simulink model "quadrotor_model"  (R2021a)
settings: Solver=VariableStepAuto  StartTime=0.0  StopTime=20  RelTol=1e-1
values from neighbouring files (symbols this model uses):
  X = [X realx(index)]    [Plot_drone_3D.m]    (also in Plot_drone_3D_sub.m)
  Y = [Y realy(index)]    [Plot_drone_3D.m]    (also in Plot_drone_3D_sub.m)
  Z = [Z realz(index)]    [Plot_drone_3D.m]    (also in Plot_drone_3D_sub.m)
undefined symbols (not defined in the file or in its folder): Discrete, Time
libraries: sm_lib x6, vrlib x2, sharedtransform x2, aerolibutil x2, nesl_utility x1, dspmtrx3 x1, ctrlSharedLib x1
settings Model: EnablePacing=on  PacingRate=10  Creator=amejiyopakapak  LastModifiedBy=user

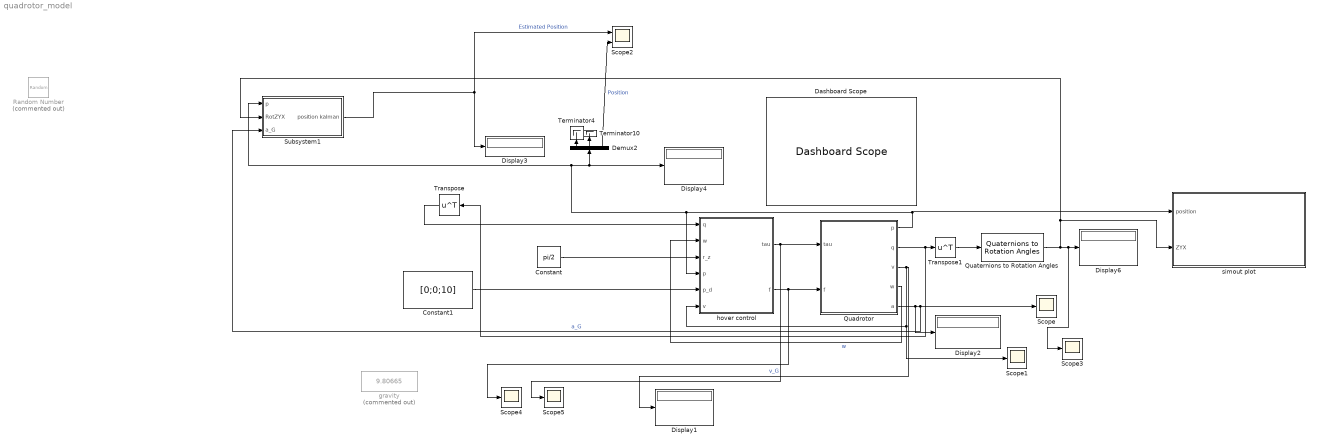
== system quadrotor_model ==
  Constant : Constant  Value=pi/2
  Constant1 : Constant  Value=[0;0;10]
  Dashboard Scope : DashboardScope
  Demux2 : Demux  Outputs=3
  Display{1..4,6} (5 alike) : Display
  Quadrotor : Subsystem
  Quaternions to Rotation Angles : sharedtransform/Quaternions to Rotation Angles  rotationOrder=ZYX  aMode=aMode
      settings: SourceProductBaseCode=AE,PW,DR,MT,UV,VE
  Random Number : RandomNumber  Commented=on  SampleTime=0.1
  Scope{,1,3..5} (5 alike) : Scope
  Scope2 : Scope  NumInputPorts=2
  Subsystem1 : Subsystem
  Terminator10 : Terminator
  Terminator4 : Terminator
  Transpose : Math  Operator=transpose  SaturateOnIntegerOverflow=on
  Transpose1 : Math  Operator=transpose  SaturateOnIntegerOverflow=on
  gravity : Constant  Commented=on  Value=9.80665
  hover control : Subsystem  mask{mass=1}
  simout plot : Subsystem
  wires:
  Quadrotor/5(a) -> Subsystem1/3(a_G), Scope/1, Display2/1  "a_G"
  Constant/1 -> hover control/3(r_z)
  Quadrotor/3(v) -> hover control/6(v), Scope1/1, Display1/1  "v_G"
  Quadrotor/2(q) -> Transpose/1, Transpose1/1
  hover control/1(tau) -> Quadrotor/1(tau), Scope5/1
  Quadrotor/4(w) -> hover control/2(w)  "w"
  Transpose/1 -> hover control/1(q)
  Quaternions to Rotation Angles/1 -> simout plot/2(ZYX), Subsystem1/2(RotZYX), Display6/1, Scope3/1
  Transpose1/1 -> Quaternions to Rotation Angles/1
  Constant1/1 -> hover control/5(p_d)
  hover control/2(f) -> Scope4/1, Quadrotor/2(f)
  Quadrotor/1(p) -> simout plot/1(position), Subsystem1/1(p), Demux2/1, Display4/1, hover control/4(p)
  Demux2/3 -> Scope2/2  "Position"
  Demux2/1 -> Terminator4/1
  Demux2/2 -> Terminator10/1
  Subsystem1/1(position kalman) -> Scope2/1, Display3/1  "Estimated Position"

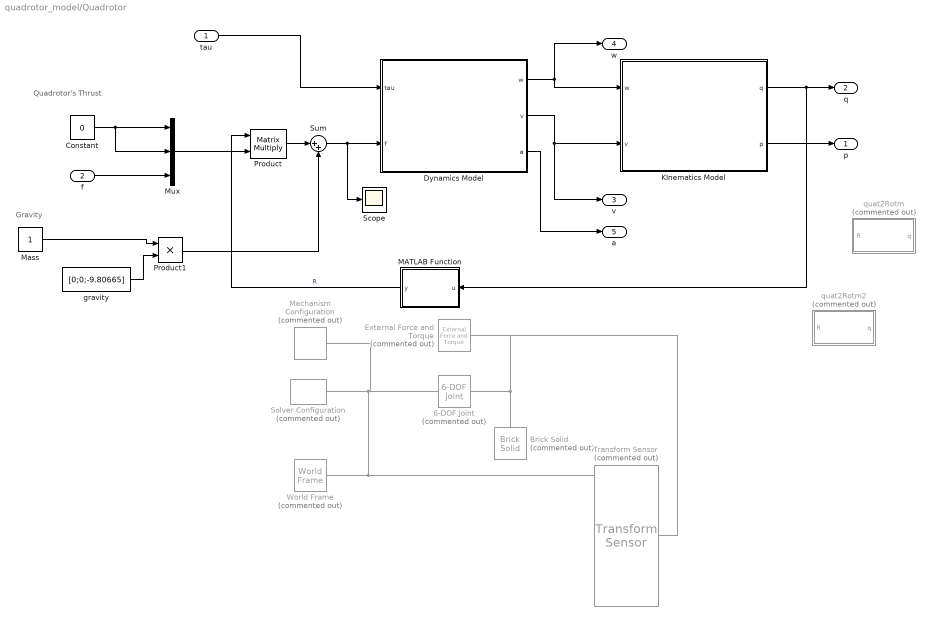
== system quadrotor_model/Quadrotor ==
  note: Quadrotor's Thrust
  note: Gravity
  tau : Inport
  f : Inport  Port=2
  6-DOF Joint : sm_lib/Joints/6-DOF Joint  Commented=on  JointMode=Normal  SenseConstraintForce=off  SenseConstraintForceX=off  SenseConstraintForceY=off  SenseConstraintForceZ=off  SenseConstraintTorque=off  SenseConstraintTorqueX=off  SenseConstraintTorqueY=off  SenseConstraintTorqueZ=off  SenseTotalForce=off  SenseTotalForceX=off  SenseTotalForceY=off  SenseTotalForceZ=off  SenseTotalTorque=off  SenseTotalTorqueX=off  SenseTotalTorqueY=off  SenseTotalTorqueZ=off  CompositeWrenchDir=FollowerOnBase  CompositeWrenchFrame=BaseFrame  PxEquilibriumPosition=0  PxEquilibriumPositionUnits=m  PxSpringStiffness=0  PxSpringStiffnessUnits=N/m  PxDampingCoefficient=0  PxDampingCoefficientUnits=N/(m/s)  PxTorqueActuationMode=NoTorque  PxMotionActuationMode=ComputedMotion  PxSensePosition=off  PxSenseVelocity=off  PxSenseAcceleration=off  PxSenseTorqueForce=off  PxSenseLowerLimitTorqueForce=off  PxSenseUpperLimitTorqueForce=off  PxLowerLimitSpecify=off  PxLowerLimitBound=-1  PxLowerLimitBoundUnits=m  PxLowerLimitStiffness=1e6  PxLowerLimitStiffnessUnits=N/m  PxLowerLimitDamping=1e3  PxLowerLimitDampingUnits=N/(m/s)  PxLowerLimitTransitionRegionWidth=1e-4  PxLowerLimitTransitionRegionWidthUnits=m  PxUpperLimitSpecify=off  PxUpperLimitBound=1  PxUpperLimitBoundUnits=m  PxUpperLimitStiffness=1e6  PxUpperLimitStiffnessUnits=N/m  PxUpperLimitDamping=1e3  PxUpperLimitDampingUnits=N/(m/s)  PxUpperLimitTransitionRegionWidth=1e-4  PxUpperLimitTransitionRegionWidthUnits=m  PxPositionTargetSpecify=off  PxPositionTargetPriority=High  PxPositionTargetValue=0  PxPositionTargetValueUnits=m  PxVelocityTargetSpecify=off  PxVelocityTargetPriority=High  PxVelocityTargetValue=0  PxVelocityTargetValueUnits=m/s  PyEquilibriumPosition=0  PyEquilibriumPositionUnits=m  PySpringStiffness=0  PySpringStiffnessUnits=N/m  PyDampingCoefficient=0  PyDampingCoefficientUnits=N/(m/s)  PyTorqueActuationMode=NoTorque  PyMotionActuationMode=ComputedMotion  PySensePosition=off  PySenseVelocity=off  PySenseAcceleration=off  PySenseTorqueForce=off  PySenseLowerLimitTorqueForce=off  PySenseUpperLimitTorqueForce=off  PyLowerLimitSpecify=off  PyLowerLimitBound=-1  PyLowerLimitBoundUnits=m  PyLowerLimitStiffness=1e6  PyLowerLimitStiffnessUnits=N/m  PyLowerLimitDamping=1e3  PyLowerLimitDampingUnits=N/(m/s)  PyLowerLimitTransitionRegionWidth=1e-4  PyLowerLimitTransitionRegionWidthUnits=m  PyUpperLimitSpecify=off  PyUpperLimitBound=1  PyUpperLimitBoundUnits=m  PyUpperLimitStiffness=1e6  PyUpperLimitStiffnessUnits=N/m  PyUpperLimitDamping=1e3  PyUpperLimitDampingUnits=N/(m/s)  PyUpperLimitTransitionRegionWidth=1e-4  PyUpperLimitTransitionRegionWidthUnits=m  PyPositionTargetSpecify=off  PyPositionTargetPriority=High  PyPositionTargetValue=0  PyPositionTargetValueUnits=m  PyVelocityTargetSpecify=off  PyVelocityTargetPriority=High  PyVelocityTargetValue=0  PyVelocityTargetValueUnits=m/s  PzEquilibriumPosition=0  PzEquilibriumPositionUnits=m  PzSpringStiffness=0  PzSpringStiffnessUnits=N/m  PzDampingCoefficient=0  PzDampingCoefficientUnits=N/(m/s)  PzTorqueActuationMode=NoTorque  PzMotionActuationMode=ComputedMotion  PzSensePosition=off  PzSenseVelocity=off  PzSenseAcceleration=off  PzSenseTorqueForce=off  PzSenseLowerLimitTorqueForce=off  PzSenseUpperLimitTorqueForce=off  PzLowerLimitSpecify=off  PzLowerLimitBound=-1  PzLowerLimitBoundUnits=m  PzLowerLimitStiffness=1e6  PzLowerLimitStiffnessUnits=N/m  PzLowerLimitDamping=1e3  PzLowerLimitDampingUnits=N/(m/s)  PzLowerLimitTransitionRegionWidth=1e-4  PzLowerLimitTransitionRegionWidthUnits=m  PzUpperLimitSpecify=off  PzUpperLimitBound=1  PzUpperLimitBoundUnits=m  PzUpperLimitStiffness=1e6  PzUpperLimitStiffnessUnits=N/m  PzUpperLimitDamping=1e3  PzUpperLimitDampingUnits=N/(m/s)  PzUpperLimitTransitionRegionWidth=1e-4  PzUpperLimitTransitionRegionWidthUnits=m  PzPositionTargetSpecify=off  PzPositionTargetPriority=High  PzPositionTargetValue=0  PzPositionTargetValueUnits=m  PzVelocityTargetSpecify=off  PzVelocityTargetPriority=High  PzVelocityTargetValue=0  PzVelocityTargetValueUnits=m/s  SphDefPosRotationMethod=None  SphDefPosRotationAngleUnits=deg  SphDefPosRotationStandardAxis=+Z  SphDefPosRotationAngle=0.0  SphDefPosRotationArbitraryAxis=[0 0 1]  SphDefPosFollAlignAxisA=+X  SphDefPosBaseAlignAxisA=+Y  SphDefPosFollAlignAxisB=+Y  SphDefPosBaseAlignAxisB=+Z  SphDefPosRotationSequenceAxes=FollowerAxes  SphDefPosRotationSequence=XYX  SphDefPosRotationSequenceAngles=[0 0 0]  SphDefPosRotationSequenceAnglesUnits=deg  SphDefPosRotationMatrix=[1 0 0; 0 1 0; 0 0 1]  SphEqPosRotationMethod=None  SphEqPosRotationAngleUnits=deg  SphEqPosRotationStandardAxis=+Z  SphEqPosRotationAngle=0.0  SphEqPosRotationArbitraryAxis=[0 0 1]  SphEqPosFollAlignAxisA=+X  SphEqPosBaseAlignAxisA=+Y  SphEqPosFollAlignAxisB=+Y  SphEqPosBaseAlignAxisB=+Z  SphEqPosRotationSequenceAxes=FollowerAxes  SphEqPosRotationSequence=XYX  SphEqPosRotationSequenceAngles=[0 0 0]  SphEqPosRotationSequenceAnglesUnits=deg  SphEqPosRotationMatrix=[1 0 0; 0 1 0; 0 0 1]  SphSpringStiffness=0  SphSpringStiffnessUnits=N*m/deg  SphDampingCoefficient=0  SphDampingCoefficientUnits=N*m/(deg/s)  SphActuateTorqueX=off  SphActuateTorqueY=off  SphActuateTorqueZ=off  SphActuateTorque=off  SphTorqueActuationMode=NoTorque  SphMotionActuationMode=ComputedMotion  SphActuationFrame=BaseFrame  SphSensePosition=off  SphSenseVelocityX=off  SphSenseVelocityY=off  SphSenseVelocityZ=off  SphSenseVelocity=off  SphSenseAccelerationX=off  SphSenseAccelerationY=off  SphSenseAccelerationZ=off  SphSenseAcceleration=off  SphSenseTorqueX=off  SphSenseTorqueY=off  SphSenseTorqueZ=off  SphSenseTorqueForce=off  SphSenseLowerLimitTorqueMag=off  SphSenseUpperLimitTorqueMag=off  SphSensingFrame=BaseFrame  SphLowerLimitSpecify=off  SphLowerLimitBound=15  SphLowerLimitBoundUnits=deg  SphLowerLimitStiffness=1e4  SphLowerLimitStiffnessUnits=N*m/deg  SphLowerLimitDamping=10  SphLowerLimitDampingUnits=N*m/(deg/s)  SphLowerLimitTransitionRegionWidth=0.1  SphLowerLimitTransitionRegionWidthUnits=deg  SphUpperLimitSpecify=off  SphUpperLimitBound=45  SphUpperLimitBoundUnits=deg  SphUpperLimitStiffness=1e4  SphUpperLimitStiffnessUnits=N*m/deg  SphUpperLimitDamping=10  SphUpperLimitDampingUnits=N*m/(deg/s)  SphUpperLimitTransitionRegionWidth=0.1  SphUpperLimitTransitionRegionWidthUnits=deg  SphPositionTargetRotationMethod=None  SphPositionTargetRotationAngleUnits=deg  SphPositionTargetRotationStandardAxis=+Z  SphPositionTargetRotationAngle=0.0  SphPositionTargetRotationArbitraryAxis=[0 0 1]  SphPositionTargetFollAlignAxisA=+X  SphPositionTargetBaseAlignAxisA=+Y  SphPositionTargetFollAlignAxisB=+Y  SphPositionTargetBaseAlignAxisB=+Z  SphPositionTargetRotationSequenceAxes=FollowerAxes  SphPositionTargetRotationSequence=XYX  SphPositionTargetRotationSequenceAngles=[0 0 0]  SphPositionTargetRotationSequenceAnglesUnits=deg  SphPositionTargetRotationMatrix=[1 0 0; 0 1 0; 0 0 1]  SphPositionTargetSpecify=off  SphPositionTargetPriority=High  SphVelocityTargetValue=[0 0 0]  SphVelocityTargetValueUnits=deg/s  SphVelocityTargetSpecify=off  SphVelocityTargetPriority=High  SphVelocityTargetInFollowerFrame=on
  Brick Solid : sm_lib/Body Elements/Brick Solid  Commented=on  GraphicAmbientColor=[0.15 0.15 0.15 1.0]  BasedOnType=Density  BrickDimensions=[1 1 1]  BrickDimensionUnits=m  CenterOfMass=[0 0 0]  CenterOfMassUnits=m  GraphicDiffuseColor=[0.5 0.5 0.5]  Density=1000  DensityUnits=kg/m^3  DoExposeReferenceFrame=on  GraphicEmissiveColor=[0.0 0.0 0.0 1.0]  ExportEntireGeometry=off  SerializedFrames=<Frames/>  MarkerShape=Sphere  MarkerSize=10  GraphicType=FromGeometry  InertiaType=CalculateFromGeometry  Mass=1  MassUnits=kg  MomentsOfInertia=[1 1 1]  MomentsOfInertiaUnits=kg*m^2  GraphicOpacity=1.0  ProductsOfInertia=[0 0 0]  ProductsOfInertiaUnits=kg*m^2  GraphicShininess=75  GraphicSpecularColor=[0.5 0.5 0.5 1.0]  GraphicVisPropType=SimpleVisualProperties
  Constant : Constant  Value=0
  Dynamics Model : Subsystem  mask{I=[1 0 0 ; 0 1 0; 0 0 1], m=1, w_0=[0;0;0], v_0=[0;0;0]}
      mask prompts: I "Body Inertia Matrix"; m "Mass"; w_0 "Initial Angular Velocity"; v_0 "Initial Linear Velocity"
      mask DialogControl Container3 Prompt: Physical Parameters
      mask DialogControl Container4 Prompt: Initial States
      mask Display: disp('Dynamics Model')
  External Force and Torque : sm_lib/Forces and Torques/External Force and Torque  Commented=on  ForceResolutionFrame=AttachedFrame  EnableForceX=off  EnableForceY=off  EnableForceZ=off  EnableForce=on  TorqueResolutionFrame=AttachedFrame  EnableTorqueX=off  EnableTorqueY=off  EnableTorqueZ=off  EnableTorque=on
  "KInematics Model " : Subsystem  mask{q_0=[1;0;0;0], p_0=[0;0;0]}
      mask prompts: q_0 "Initial Orienetation (in quaternion)"; p_0 "Initial Position"
      mask DialogControl Container3 Prompt: Initial States
      mask Display: disp('Kinematics Model')
  MATLAB Function : MATLAB Function  TreatAsAtomicUnit=on
  Mass : Constant
  Mechanism Configuration : sm_lib/Utilities/Mechanism Configuration  Commented=on  UniformGravity=Constant  GravityVector=[0 0 -9.80665]  GravityVectorUnits=m/s^2  GravityUnits=m/s^2  LinearizationDelta=0.001  JointModeTransitionNonlinearIterations=2
  Mux : Mux  Inputs=3
  Product : Product  Multiplication=Matrix(*)
  Product1 : Product
  Scope : Scope
  Solver Configuration : nesl_utility/Solver Configuration  Commented=on  PhysicalDomain=network_engine_domain  SubClassName=solver  LeftPortType=input  RightPortType=generic  Tones=[]  Harmonics=[]  SimulateNoise=off  Profile=off  UseLocalSampling=off  EnableSwitchedLinearOptims=on  FrequencyDomain=off  UseCCode=off  RelTol=0.001  AbsTol=1e-06  MinStep=1e-09  ToWorkspace=off  RevertToSquareIcSolve=off  NumHomotopyIterations=100  PhasorMode=off  PhasorModeNumHarmonics=1  DoDC=off  ResidualTolerance=1e-09  UseLocalSolver=off  LocalSolverChoice=NE_BACKWARD_EULER_ADVANCER  LocalSolverSampleTime=0.001  DoFixedCost=off  MaxNonlinIter=3  MaxModeIter=2  ComputeImpulses=off  ImpulseIterations=2  LinearAlgebra=auto  EquationFormulation=NE_TIME_EF  DelaysMemoryBudget=1024  AutomaticFiltering=on  FilteringTimeConstant=0.001  PartitionStorageMethod=AS_NEEDED  PartitionMemoryBudget=1024  PartitionMethod=ROBUST
  Sum : Sum  Inputs=|++
  Transform Sensor : sm_lib/Frames and Transforms/Transform Sensor  Commented=on  MeasurementFrame=World  SenseAngle=off  SenseAxis=off  SenseAngle1=off  SenseAngle2=off  SenseAngle3=off  SenseQ=on  SenseR=off  SenseOmegaX=on  SenseOmegaY=on  SenseOmegaZ=on  SenseOmega1=off  SenseOmega2=off  SenseOmega3=off  SenseQDot=off  SenseRDot=off  SenseAlphaX=off  SenseAlphaY=off  SenseAlphaZ=off  SenseAlpha1=off  SenseAlpha2=off  SenseAlpha3=off  SenseQDDot=off  SenseRDDot=off  SenseX=on  SenseY=on  SenseZ=on  SenseRad=off  SenseAzim=off  SenseDist=off  SenseInc=off  SenseXDot=on  SenseYDot=on  SenseZDot=on  SenseRadDot=off  SenseAzimDot=off  SenseDistDot=off  SenseIncDot=off  SenseXDDot=off  SenseYDDot=off  SenseZDDot=off  SenseRadDDot=off  SenseAzimDDot=off  SenseDistDDot=off  SenseIncDDot=off
  World Frame : sm_lib/Frames and Transforms/World Frame  Commented=on
  gravity : Constant  Value=[0;0;-9.80665]
  quat2Rotm : Subsystem  Commented=on
      mask Display: disp('R(q)')
  quat2Rotm2 : Subsystem  Commented=on
      mask Display: disp('R(q)')
  p : Outport
  q : Outport  Port=2
  v : Outport  Port=3
  w : Outport  Port=4
  a : Outport  Port=5
  wires:
  Dynamics Model/1(w) -> "KInematics Model "/1(w), w/1
  "KInematics Model "/2(p) -> p/1
  Dynamics Model/2(v) -> v/1, "KInematics Model "/2(v)
  f/1 -> Mux/3
  Constant/1 -> Mux/2, Mux/1
  Product/1 -> Sum/1
  Product1/1 -> Sum/2
  gravity/1 -> Product1/2
  Mass/1 -> Product1/1
  Dynamics Model/3(a) -> a/1
  MATLAB Function/1(y) -> Product/1  "R"
  Mux/1 -> Product/2
  Sum/1 -> Scope/1, Dynamics Model/2(f)
  tau/1 -> Dynamics Model/1(tau)
  "KInematics Model "/1(q) -> MATLAB Function/1(u), q/1
  connections:
  Solver Configuration/RConn1 -- Mechanism Configuration/RConn1 -- 6-DOF Joint/LConn1 -- Transform Sensor/RConn1 -- World Frame/RConn1
  6-DOF Joint/RConn1 -- External Force and Torque/RConn1 -- Transform Sensor/LConn1 -- Brick Solid/RConn1

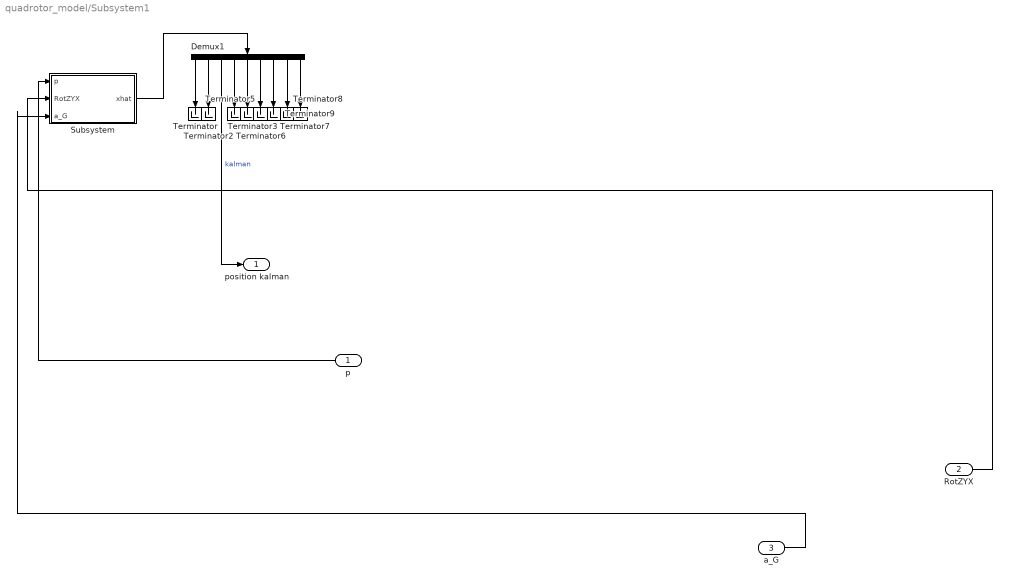
== system quadrotor_model/Subsystem1 ==
  p : Inport
  RotZYX : Inport  Port=2
  a_G : Inport  Port=3
  Demux1 : Demux  Outputs=9
  Subsystem : Subsystem
  Terminator{,2..3,5..9} (8 alike) : Terminator
  position kalman : Outport
  wires:
  Demux1/5 -> Terminator5/1
  Demux1/1 -> Terminator/1
  Demux1/8 -> Terminator7/1
  Demux1/4 -> Terminator3/1
  Demux1/9 -> Terminator8/1
  Demux1/6 -> Terminator6/1
  Demux1/7 -> Terminator9/1
  Demux1/2 -> Terminator2/1
  RotZYX/1 -> Subsystem/2(RotZYX)
  Subsystem/1(xhat) -> Demux1/1
  Demux1/3 -> position kalman/1  "kalman"
  p/1 -> Subsystem/1(p)
  a_G/1 -> Subsystem/3(a_G)

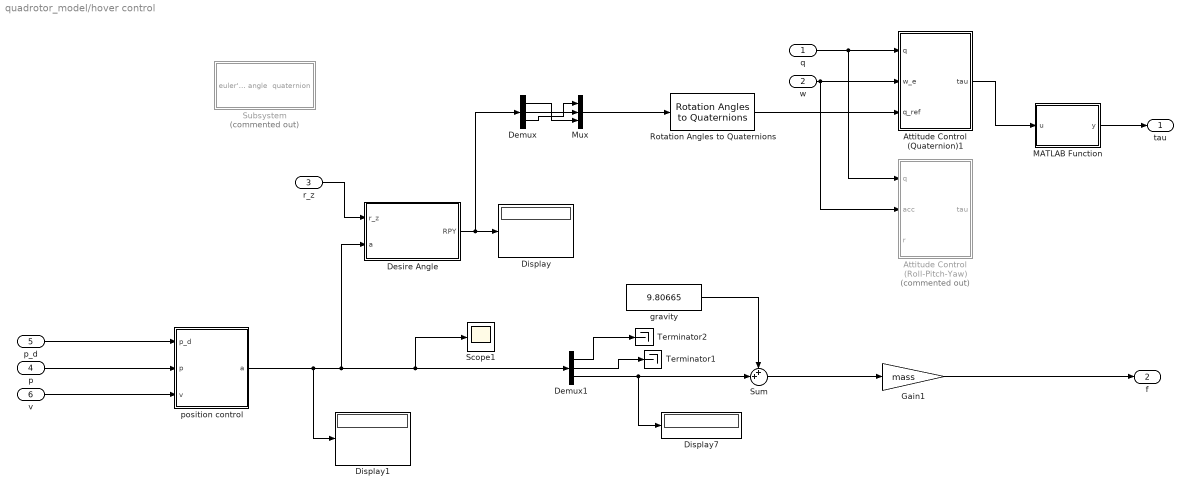
== system quadrotor_model/hover control ==
  q : Inport
  w : Inport  Port=2
  r_z : Inport  Port=3
  p : Inport  Port=4
  p_d : Inport  Port=5
  v : Inport  Port=6
  Attitude Control (Quaternion)1 : Subsystem  mask{K_q=150*diag([1;1;1]), K_w=50*diag([1;1;1])}
      mask prompts: K_q "Proportional Gain"; K_w "Velocity Gain"
      mask DialogControl Container3 Prompt: Control Gain
  Attitude Control (Roll-Pitch-Yaw) : Subsystem  Commented=on
  Demux : Demux  Outputs=3
  Demux1 : Demux  Outputs=3
  Desire Angle : Subsystem
  Display : Display
  Display1 : Display
  Display7 : Display
  Gain1 : Gain  Gain=mass
  MATLAB Function : MATLAB Function  TreatAsAtomicUnit=on
  Mux : Mux  Inputs=3
  Rotation Angles to Quaternions : sharedtransform/Rotation Angles to Quaternions  rotationOrder=ZYX  aMode=aMode
      settings: SourceProductBaseCode=AE,PW,DR,MT,UV,VE
  Scope1 : Scope
  Subsystem : Subsystem  Commented=on
  Sum : Sum  Inputs=++|
  Terminator1 : Terminator
  Terminator2 : Terminator
  gravity : Constant  Value=9.80665  VectorParams1D=off
  position control : Subsystem  mask{K_p=2*diag([1;1;1]), K_d=1*diag([1;1;1]), K_i=0*diag([1;1;1])}
  tau : Outport  SampleTime=1/100
  f : Outport  Port=2  SampleTime=1/100
  wires:
  q/1 -> Attitude Control (Quaternion)1/1(q), Attitude Control (Roll-Pitch-Yaw)/1(q)
  Rotation Angles to Quaternions/1 -> Attitude Control (Quaternion)1/3(q_ref)
  Demux1/2 -> Terminator1/1
  Sum/1 -> Gain1/1
  Demux1/3 -> Display7/1, Sum/2
  MATLAB Function/1(y) -> tau/1
  Attitude Control (Quaternion)1/1(tau) -> MATLAB Function/1(u)
  gravity/1 -> Sum/1
  Demux1/1 -> Terminator2/1
  Mux/1 -> Rotation Angles to Quaternions/1
  w/1 -> Attitude Control (Quaternion)1/2(w_e), Attitude Control (Roll-Pitch-Yaw)/2(acc)
  v/1 -> position control/3(v)
  r_z/1 -> Desire Angle/1(r_z)
  p_d/1 -> position control/1(p_d)
  p/1 -> position control/2(p)
  position control/1(a) -> Scope1/1, Demux1/1, Desire Angle/2(a), Display1/1
  Gain1/1 -> f/1
  Demux/2 -> Mux/2
  Demux/1 -> Mux/3
  Demux/3 -> Mux/1
  Desire Angle/1(RPY) -> Demux/1, Display/1

== system quadrotor_model/simout plot ==
  position : Inport
  ZYX : Inport  Port=2
  Clock : Clock
  To Workspace : ToWorkspace  VariableName=ZYX  SampleTime=0.05
      settings: Save2DSignal=2-D array (concatenate along first dimension)
  To Workspace1 : ToWorkspace  VariableName=position  SampleTime=0.05
  To Workspace2 : ToWorkspace  VariableName=time  SampleTime=0.05
      settings: Save2DSignal=2-D array (concatenate along first dimension)
  wires:
  ZYX/1 -> To Workspace/1
  position/1 -> To Workspace1/1
  Clock/1 -> To Workspace2/1

== system quadrotor_model/Quadrotor/Dynamics Model ==
  tau : Inport  PortDimensions=3
  f : Inport  Port=2  PortDimensions=3
  Initial Angular Velocity : Constant  Value=w_0
  Initial Linear Velocity : Constant  Value=v_0
  Integrator3 : Integrator  InitialConditionSource=external
  Integrator4 : Integrator  InitialConditionSource=external
  Orientation Dynamics : Subsystem  mask{I=I}
      mask prompts: I "Body Inertia Matrix"
      settings: PortSchema="{\"entries\":[{\"content\":{\"sides\":[{\"content\":{\"connectorIds\":[\"In1\"]},\"type\":\"ConnectorPlacement.EquallySpacedRectSide\",\"uuid\":\"c0bebf24-b4c5-4120-b4bc-e257700e30ac\"},{\"content\":{\"connectorIds\":[\"In2\",\"Out1\"],\"side\":\"RIGHT\"},\"type\":\"ConnectorPlacement.EquallySpacedRectSide\",\"uuid\":\"4f6c7abb-67af-4a33-8fe1-31c16aba2e01\"},{\"content\":{\"connectorIds\":[],\"side\":\"TOP\"},\"type\":\"ConnectorPlacement.EquallySpacedRectSide\",\"uuid\":\"8bb59cb6-0e62-4460-a924-40655b1bfaef\"},{\"content\":{\"connectorIds\":[],\"side\":\"HIDDEN\"},\"type\":\"ConnectorPlacement.EquallySpacedRectSide\",\"uuid\":\"077b0ca6-0b74-4b7e-aec6-ebc5a9681944\"}]},\"type\":\"ConnectorPlacement.EquallySpacedConnector\",\"uuid\":\"b5fc50ba-032b-41ac-a5ea-9388df4800bf\"}],\"packageUris\":[\"http://schema.mathworks.com/mf0/Connector/R2020b\"],\"version\":\"1.0\"}"
      mask DialogControl Container3 Prompt: Physical Parameter
      mask Display: disp('Orientation Dynamics')
  Position Dynamics : Subsystem  mask{m=m}
      mask prompts: m "Mass"
      mask DialogControl Container3 Prompt: Physical Parameter
      mask Display: disp('Position Dynamics')
  w : Outport
  v : Outport  Port=2
  a : Outport  Port=3
  wires:
  tau/1 -> Orientation Dynamics/1(tau)
  Integrator3/1 -> Orientation Dynamics/2(w), w/1  "w"
  Position Dynamics/1(dv) -> a/1, Integrator4/1
  Initial Linear Velocity/1 -> Integrator4/2
  Orientation Dynamics/1(dw) -> Integrator3/1
  Integrator4/1 -> v/1  "v"
  f/1 -> Position Dynamics/1(f)
  Initial Angular Velocity/1 -> Integrator3/2

== system quadrotor_model/Quadrotor/KInematics Model  ==
  w : Inport
  v : Inport  Port=2
  Initial Orientation : Constant  Value=q_0
  Initial Position : Constant  Value=p_0
  Integrator1 : Integrator  InitialConditionSource=external
  Integrator2 : Integrator  InitialConditionSource=external
  Orientation Kinematics : Subsystem
      settings: PortSchema="{\"entries\":[{\"content\":{\"sides\":[{\"content\":{\"connectorIds\":[\"In1\"]},\"type\":\"ConnectorPlacement.EquallySpacedRectSide\",\"uuid\":\"c0bebf24-b4c5-4120-b4bc-e257700e30ac\"},{\"content\":{\"connectorIds\":[\"In2\",\"Out1\"],\"side\":\"RIGHT\"},\"type\":\"ConnectorPlacement.EquallySpacedRectSide\",\"uuid\":\"4f6c7abb-67af-4a33-8fe1-31c16aba2e01\"},{\"content\":{\"connectorIds\":[],\"side\":\"TOP\"},\"type\":\"ConnectorPlacement.EquallySpacedRectSide\",\"uuid\":\"8bb59cb6-0e62-4460-a924-40655b1bfaef\"},{\"content\":{\"connectorIds\":[],\"side\":\"HIDDEN\"},\"type\":\"ConnectorPlacement.EquallySpacedRectSide\",\"uuid\":\"077b0ca6-0b74-4b7e-aec6-ebc5a9681944\"}]},\"type\":\"ConnectorPlacement.EquallySpacedConnector\",\"uuid\":\"b5fc50ba-032b-41ac-a5ea-9388df4800bf\"}],\"packageUris\":[\"http://schema.mathworks.com/mf0/Connector/R2020b\"],\"version\":\"1.0\"}"
  Position Kinematics : Subsystem
  Vector Normalization : Subsystem
      mask Display: disp('v''=v/|v|')
  q : Outport
  p : Outport  Port=2
  wires:
  Position Kinematics/1(dp) -> Integrator2/1
  Orientation Kinematics/1(dq) -> Integrator1/1
  Integrator1/1 -> Vector Normalization/1(v)
  Integrator2/1 -> p/1  "p"
  Initial Position/1 -> Integrator2/2
  Initial Orientation/1 -> Integrator1/2
  w/1 -> Orientation Kinematics/1(w)
  Vector Normalization/1(v') -> Orientation Kinematics/2(q), q/1  "q"
  v/1 -> Position Kinematics/1(v)

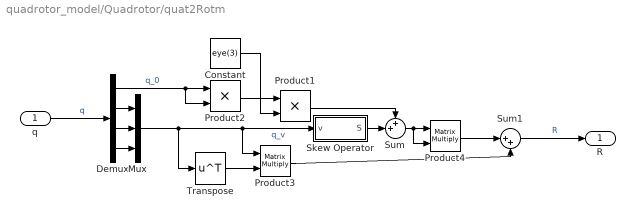
== system quadrotor_model/Quadrotor/quat2Rotm ==
  q : Inport
  Constant : Constant  Value=eye(3)
  Demux : Demux
  Mux : Mux  Inputs=3
  Product1 : Product
  Product2 : Product
  Product3 : Product  Multiplication=Matrix(*)
  Product4 : Product  Multiplication=Matrix(*)
  Skew Operator : Subsystem  Description=S(v)
      mask Display: disp('S(v)')
  Sum : Sum  Inputs=++|
  Sum1 : Sum  Inputs=|++
  Transpose : Math  Operator=transpose  SaturateOnIntegerOverflow=on
  R : Outport
  wires:
  q/1 -> Demux/1  "q"
  Sum1/1 -> R/1  "R"
  Mux/1 -> Transpose/1, Product3/1, Skew Operator/1(v)  "q_v"
  Sum/1 -> Product4/1, Product4/2
  Demux/1 -> Product2/2, Product2/1  "q_0"
  Transpose/1 -> Product3/2
  Demux/2 -> Mux/1
  Demux/3 -> Mux/2
  Demux/4 -> Mux/3
  Product4/1 -> Sum1/1
  Constant/1 -> Product1/2
  Product2/1 -> Product1/1
  Skew Operator/1(S) -> Sum/2
  Product1/1 -> Sum/1
  Product3/1 -> Sum1/2

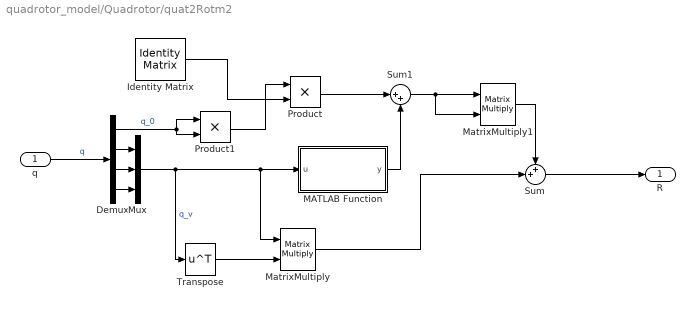
== system quadrotor_model/Quadrotor/quat2Rotm2 ==
  q : Inport
  Demux : Demux
  Identity Matrix : dspmtrx3/Identity Matrix  Inherit=off  N=3  Ts=1  dataType=double  isSigned=on  wordLen=16  udDataType=sfix(16)  fracBitsMode=Best precision  numFracBits=15  OutDataTypeStr=double  LastOutDataTypeStr=double
  MATLAB Function : MATLAB Function  TreatAsAtomicUnit=on
  MatrixMultiply : Product  Multiplication=Matrix(*)
  MatrixMultiply1 : Product  Multiplication=Matrix(*)
  Mux : Mux  Inputs=3
  Product : Product
  Product1 : Product
  Sum : Sum  Inputs=++|
  Sum1 : Sum  Inputs=|++
  Transpose : Math  Operator=transpose  SaturateOnIntegerOverflow=on
  R : Outport
  wires:
  q/1 -> Demux/1  "q"
  Mux/1 -> Transpose/1, MatrixMultiply/1, MATLAB Function/1(u)  "q_v"
  Demux/1 -> Product1/2, Product1/1  "q_0"
  Demux/2 -> Mux/1
  Demux/3 -> Mux/2
  Demux/4 -> Mux/3
  Identity Matrix/1 -> Product/2
  Product/1 -> Sum1/1
  MATLAB Function/1(y) -> Sum1/2
  Transpose/1 -> MatrixMultiply/2
  MatrixMultiply/1 -> Sum/2
  Sum/1 -> R/1
  Sum1/1 -> MatrixMultiply1/2, MatrixMultiply1/1
  MatrixMultiply1/1 -> Sum/1
  Product1/1 -> Product/1

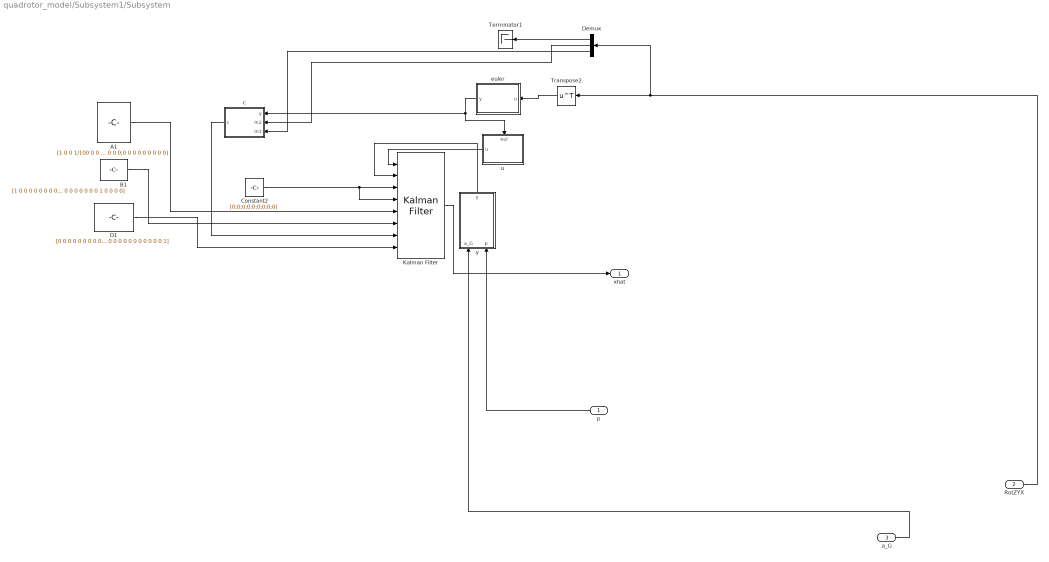
== system quadrotor_model/Subsystem1/Subsystem ==
  p : Inport
  RotZYX : Inport  Port=2
  a_G : Inport  Port=3
  A1 : Constant  Value=[1 0 0 1/100 0 0 0 0 0;0 1 0 0 1/100 0 0 0 0;0 0 1 0 0 1/100 0 0 0;0 0 0 1 0 0 0 0 0;0 0 0 0 1 0 0 0 0;0 0 0 0 0 1 0 0 0;0 0 0 0 0 0 0 0 0;0 0 0 0 0 0 0 0 0;0 0 0 0 0 0 0 0 0]  SampleTime=1/100
  B1 : Constant  Value=[1 0 0 0 0 0 0 0 0 0 0 0 0;0 1 0 0 0 0 0 0 0 0 0 0 0;0 0 1 0 0 0 0 0 0 0 0 0 0;0 0 0 1 0 0 0 0 0 0 0 0 0;0 0 0 0 1 0 0 0 0 0 0 0 0;0 0 0 0 0 1 0 0 0 0 0 0 0;0 0 0 0 0 0 1 0 0 0 0 0 0;0 0 0 0 0 0 0 1 0 0 0 0 0;0 0 0 0 0 0 0 0 1 0 0 0 0]  SampleTime=1/100
  Constant2 : Constant  Value=[0;0;0;0;0;0;0;0;0]
  D1 : Constant  Value=[0 0 0 0 0 0 0 0 0 1 0 0 0;0 0 0 0 0 0 0 0 0 0 1 0 0;0 0 0 0 0 0 0 0 0 0 0 1 0;0 0 0 0 0 0 0 0 0 0 0 0 1]  SampleTime=1/100
  Demux : Demux  Outputs=3
  Kalman Filter : ctrlSharedLib/Kalman Filter  TimeDomain=Discrete-Time  UseCurrentEstimator=on  ModelSource=Input port  ModelSourceVariable=ss(0.95,1,1,0,1)  A=0.95  B=1  C=1  D=0  NumberOfStates=9  NumberOfInputs=13  NumberOfOutputs=4  InitialEstimateSource=Input port  X0=0  P0=10  UseK=off  UseGH=on  NumberOfProcessNoiseInputs=1  G=[0;0;1/10000;0;0;1/100;0;0;1]  TimeInvariantG=on  H=[0;0;0;0]  TimeInvariantH=on  Q=0.0898  TimeInvariantQ=on  R=diag([0.1,0.1,0.1,0.008])  TimeInvariantR=on  N=[0,0,0,0]  TimeInvariantN=on  AddInputPort=on  AddEnablePort=off  OutputEstimatedY=off  OutputP=off  Ts=1/100
  Terminator1 : Terminator
  Transpose2 : Math  Operator=transpose  SaturateOnIntegerOverflow=on
  c : Subsystem
  euler : MATLAB Function  TreatAsAtomicUnit=on
  u : Subsystem
      settings: PortSchema="{\"entries\":[{\"content\":{\"sides\":[{\"content\":{\"connectorIds\":[]},\"type\":\"ConnectorPlacement.EquallySpacedRectSide\",\"uuid\":\"26540b1e-a89b-4888-9ec4-fd7f7f630feb\"},{\"content\":{\"connectorIds\":[\"Out1\"],\"side\":\"RIGHT\"},\"type\":\"ConnectorPlacement.EquallySpacedRectSide\",\"uuid\":\"c38f773a-f816-4bcf-adbb-33b029198f6a\"},{\"content\":{\"connectorIds\":[\"In1\"],\"side\":\"TOP\"},\"type\":\"ConnectorPlacement.EquallySpacedRectSide\",\"uuid\":\"b3e9f8ed-a140-475e-aa7e-f57dd0c447f1\"}]},\"type\":\"ConnectorPlacement.EquallySpacedConnector\",\"uuid\":\"be05692c-b490-4b4e-9a7a-7a384c24560c\"}],\"packageUris\":[\"http://schema.mathworks.com/mf0/Connector/R2020b\"],\"version\":\"1.0\"}"
  y : Subsystem
  xhat : Outport
  wires:
  Transpose2/1 -> euler/1(u)
  RotZYX/1 -> Demux/1, Transpose2/1
  Constant2/1 -> Kalman Filter/4, Kalman Filter/3
  A1/1 -> Kalman Filter/5
  D1/1 -> Kalman Filter/8
  B1/1 -> Kalman Filter/6
  c/1(c) -> Kalman Filter/7
  euler/1(y) -> c/1(y), u/1(eul)
  Demux/2 -> c/2(In2)
  u/1(u) -> Kalman Filter/1
  Demux/1 -> Terminator1/1
  Kalman Filter/1 -> xhat/1
  y/1(y) -> Kalman Filter/2
  Demux/3 -> c/3(In3)
  p/1 -> y/2(p)
  a_G/1 -> y/1(a_G)

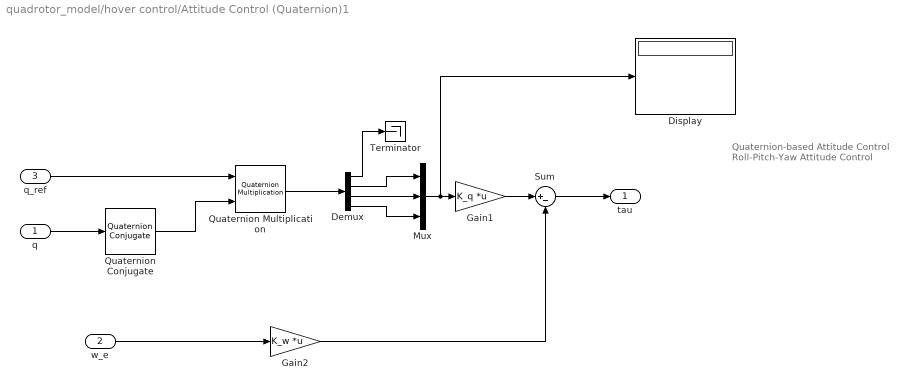
== system quadrotor_model/hover control/Attitude Control (Quaternion)1 ==
  note: Quaternion-based Attitude Control
      | Roll-Pitch-Yaw Attitude Control
  q : Inport
  w_e : Inport  Port=2
  q_ref : Inport  Port=3
  Demux : Demux
  Display : Display
  Gain1 : Gain  Gain=K_q  Multiplication=Matrix(K*u)
  Gain2 : Gain  Gain=K_w  Multiplication=Matrix(K*u)
  Mux : Mux  Inputs=3
  Quaternion Conjugate : aerolibutil/Quaternion Conjugate
      settings: SourceProductBaseCode=AE
  Quaternion Multiplication : aerolibutil/Quaternion Multiplication
  Sum : Sum  Inputs=|+-
  Terminator : Terminator
  tau : Outport
  wires:
  w_e/1 -> Gain2/1
  Quaternion Conjugate/1 -> Quaternion Multiplication/2
  Sum/1 -> tau/1
  Mux/1 -> Display/1, Gain1/1
  Gain2/1 -> Sum/2
  Gain1/1 -> Sum/1
  Demux/1 -> Terminator/1
  Demux/3 -> Mux/2
  Demux/4 -> Mux/3
  Demux/2 -> Mux/1
  Quaternion Multiplication/1 -> Demux/1
  q_ref/1 -> Quaternion Multiplication/1
  q/1 -> Quaternion Conjugate/1

== system quadrotor_model/hover control/Attitude Control (Roll-Pitch-Yaw) ==
  note: Quaternion-based Attitude Control
      | Roll-Pitch-Yaw Attitude Control
  q : Inport
  acc : Inport  Port=2
  r : Inport  Port=3
  tau : Outport
  wires:
  ? -> tau/1

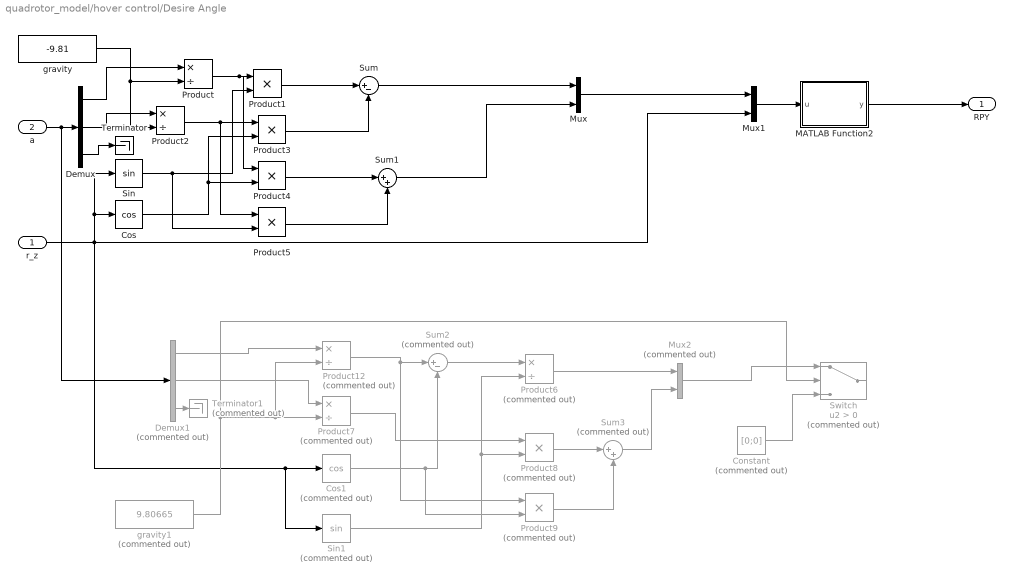
== system quadrotor_model/hover control/Desire Angle ==
  r_z : Inport
  a : Inport  Port=2
  Constant : Constant  Commented=on  Value=[0;0]
  Cos : Trigonometry  Operator=cos
  Cos1 : Trigonometry  Commented=on  Operator=cos
  Demux : Demux  Outputs=3
  Demux1 : Demux  Commented=on  Outputs=3
  MATLAB Function2 : MATLAB Function  TreatAsAtomicUnit=on
  Mux : Mux  Inputs=2
  Mux1 : Mux  Inputs=2
  Mux2 : Mux  Commented=on  Inputs=2
  Product : Product  Inputs=*/
  Product{1,3..5} (4 alike) : Product
  Product12 : Product  Commented=on  Inputs=*/
  Product2 : Product  Inputs=*/
  Product6 : Product  Commented=on  Inputs=*/
  Product7 : Product  Commented=on  Inputs=*/
  Product8 : Product  Commented=on
  Product9 : Product  Commented=on
  Sin : Trigonometry
  Sin1 : Trigonometry  Commented=on
  Sum : Sum  Inputs=|+-
  Sum1 : Sum  Inputs=|++
  Sum2 : Sum  Commented=on  Inputs=|+-
  Sum3 : Sum  Commented=on  Inputs=|++
  Switch : Switch  Commented=on  Criteria=u2 > Threshold
  Terminator : Terminator
  Terminator1 : Terminator  Commented=on
  gravity : Constant  Value=-9.81  VectorParams1D=off
  gravity1 : Constant  Commented=on  Value=9.80665  VectorParams1D=off
  RPY : Outport
  wires:
  Mux1/1 -> MATLAB Function2/1(u)
  Demux/1 -> Product/1
  gravity/1 -> Product/2, Product2/2
  Product/1 -> Product4/1, Product1/1
  Sin/1 -> Product5/2, Product1/2
  Product1/1 -> Sum/1
  Demux/2 -> Product2/1
  Product2/1 -> Product5/1, Product3/1
  Cos/1 -> Product4/2, Product3/2
  Product3/1 -> Sum/2
  Sum/1 -> Mux/1
  Product4/1 -> Sum1/1
  Product5/1 -> Sum1/2
  Sum1/1 -> Mux/2
  Demux/3 -> Terminator/1
  a/1 -> Demux1/1, Demux/1
  r_z/1 -> Sin1/1, Cos1/1, Mux1/2, Sin/1, Cos/1
  Demux1/1 -> Product12/1
  Product12/1 -> Product9/1, Sum2/1
  Cos1/1 -> Product9/2, Sum2/2
  Sum2/1 -> Product6/1
  Sin1/1 -> Product8/2, Product6/2
  Product6/1 -> Mux2/1
  MATLAB Function2/1(y) -> RPY/1
  Demux1/2 -> Product7/1
  Product7/1 -> Product8/1
  Product8/1 -> Sum3/1
  Product9/1 -> Sum3/2
  Sum3/1 -> Mux2/2
  gravity1/1 -> Switch/2, Product7/2, Product12/2
  Mux2/1 -> Switch/1
  Constant/1 -> Switch/3
  Demux1/3 -> Terminator1/1
  Mux/1 -> Mux1/1

== system quadrotor_model/hover control/Subsystem ==
  euler's angle : Inport
  MATLAB Function : MATLAB Function  TreatAsAtomicUnit=on
  quaternion : Outport
  wires:
  MATLAB Function/1(q) -> quaternion/1
  euler's angle/1 -> MATLAB Function/1(r)

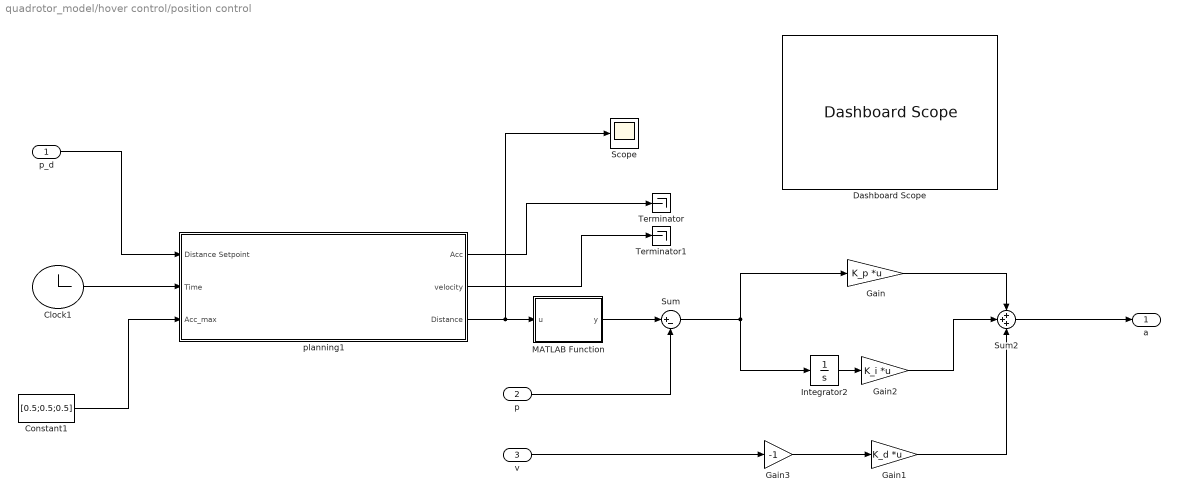
== system quadrotor_model/hover control/position control ==
  p_d : Inport
  p : Inport  Port=2
  v : Inport  Port=3
  Clock1 : Clock
  Constant1 : Constant  Value=[0.5;0.5;0.5]
  Dashboard Scope : DashboardScope
  Gain : Gain  Gain=K_p  Multiplication=Matrix(K*u)
  Gain1 : Gain  Gain=K_d  Multiplication=Matrix(K*u)
  Gain2 : Gain  Gain=K_i  Multiplication=Matrix(K*u)
  Gain3 : Gain  Gain=-1
  Integrator2 : Integrator
  MATLAB Function : MATLAB Function  TreatAsAtomicUnit=on
  Scope : Scope
  Sum : Sum  Inputs=|+-
  Sum2 : Sum  Inputs=+++
  Terminator : Terminator
  Terminator1 : Terminator
  planning1 : Subsystem
  a : Outport
  wires:
  Constant1/1 -> planning1/3(Acc_max)
  Sum2/1 -> a/1
  p/1 -> Sum/2
  planning1/1("Acc ") -> Terminator/1
  planning1/2(velocity) -> Terminator1/1
  Sum/1 -> Gain/1, Integrator2/1
  Gain/1 -> Sum2/1
  v/1 -> Gain3/1
  Gain3/1 -> Gain1/1
  Gain1/1 -> Sum2/3
  Integrator2/1 -> Gain2/1
  Gain2/1 -> Sum2/2
  p_d/1 -> planning1/1(Distance Setpoint)
  MATLAB Function/1(y) -> Sum/1
  planning1/3(Distance) -> Scope/1, MATLAB Function/1(u)
  Clock1/1 -> planning1/2(Time)

== system quadrotor_model/Quadrotor/Dynamics Model/Orientation Dynamics ==
  tau : Inport
  w : Inport  Port=2
  Body Inertia Matrix : Constant  Value=I
  Cross Product : vrlib/Utilities/Cross Product
  Matrix Multiply : Product  Multiplication=Matrix(*)
  Product : Product  Inputs=/*  Multiplication=Matrix(*)  OutDataTypeStr=Inherit: Inherit via back propagation
  Sum : Sum  Inputs=+-|
  dw : Outport
  wires:
  Body Inertia Matrix/1 -> Product/1, Matrix Multiply/1
  Matrix Multiply/1 -> Cross Product/2
  w/1 -> Cross Product/1, Matrix Multiply/2
  Cross Product/1 -> Sum/2
  tau/1 -> Sum/1
  Sum/1 -> Product/2
  Product/1 -> dw/1

== system quadrotor_model/Quadrotor/Dynamics Model/Position Dynamics ==
  f : Inport
  Mass : Constant  Value=m
  Product1 : Product  Inputs=*/
  dv : Outport
  wires:
  Product1/1 -> dv/1
  f/1 -> Product1/1
  Mass/1 -> Product1/2

== system quadrotor_model/Quadrotor/KInematics Model /Orientation Kinematics ==
  w : Inport
  q : Inport  Port=2
  Cross Product : vrlib/Utilities/Cross Product
  Demux : Demux
  Dot Product : DotProduct  InputSameDT=on  OutDataTypeStr=Inherit: Inherit via internal rule
  Gain1 : Gain  Gain=-1
  Mux : Mux  Inputs=3
  Mux1 : Mux  Inputs=2
  Product : Product
  Sum : Sum  Inputs=|++
  dq : Outport
  wires:
  q/1 -> Demux/1  "q"
  Demux/2 -> Mux/1
  Demux/3 -> Mux/2
  w/1 -> Product/2, Dot Product/2, Cross Product/2  "w"
  Demux/4 -> Mux/3
  Mux/1 -> Dot Product/1, Cross Product/1  "q_v"
  Mux1/1 -> dq/1
  Demux/1 -> Product/1  "q_0"
  Product/1 -> Sum/1
  Cross Product/1 -> Sum/2
  Sum/1 -> Mux1/2
  Dot Product/1 -> Gain1/1
  Gain1/1 -> Mux1/1

== system quadrotor_model/Quadrotor/KInematics Model /Position Kinematics ==
  v : Inport
  dp : Outport
  wires:
  v/1 -> dp/1

== system quadrotor_model/Quadrotor/KInematics Model /Vector Normalization ==
  v : Inport
  Dot Product1 : DotProduct  InputSameDT=on  OutDataTypeStr=Inherit: Inherit via internal rule
  Product3 : Product  Inputs=*/
  Sqrt : Sqrt  SaturateOnIntegerOverflow=on
  v' : Outport
  wires:
  Product3/1 -> v'/1
  v/1 -> Dot Product1/2, Product3/1, Dot Product1/1
  Dot Product1/1 -> Sqrt/1
  Sqrt/1 -> Product3/2

== system quadrotor_model/Quadrotor/quat2Rotm/Skew Operator ==
  v : Inport
  Constant : Constant  Value=0
  Demux1 : Demux  Outputs=3
  Demux2 : Demux  Outputs=3
  Gain1 : Gain  Gain=-1
  Matrix Concatenate : Concatenate  NumInputs=3  Mode=Multidimensional array  ConcatenateDimension=2
  Mux1 : Mux  Inputs=3
  Mux2 : Mux  Inputs=3
  Mux3 : Mux  Inputs=3
  S : Outport
  wires:
  Constant/1 -> Mux3/3, Mux2/2, Mux1/1
  Demux1/3 -> Mux1/2
  Matrix Concatenate/1 -> S/1
  Demux1/1 -> Mux2/3
  v/1 -> Demux1/1, Gain1/1  "v"
  Demux2/1 -> Mux3/2
  Mux3/1 -> Matrix Concatenate/3
  Gain1/1 -> Demux2/1
  Demux2/3 -> Mux2/1
  Mux1/1 -> Matrix Concatenate/1
  Demux2/2 -> Mux1/3
  Demux1/2 -> Mux3/1
  Mux2/1 -> Matrix Concatenate/2

== system quadrotor_model/Subsystem1/Subsystem/c ==
  y : Inport
  In2 : Inport  Port=2
  In3 : Inport  Port=3
  Constant : Constant
  Constant1 : Constant  Value=0
  Cos : Trigonometry  Operator=cos
  Cos1 : Trigonometry  Operator=cos
  Divide : Product  Inputs=**
  Divide1 : Product  Inputs=*/
  MATLAB Function : MATLAB Function  TreatAsAtomicUnit=on
  Mux : Mux  Inputs=36
  Reshape : Reshape  OutputDimensionality=Customize  OutputDimensions=[4,9]
  c : Outport  SampleTime=1/100
  wires:
  In2/1 -> Cos/1
  In3/1 -> Cos1/1
  Cos/1 -> Divide/1
  Cos1/1 -> Divide/2
  Constant/1 -> Divide1/1
  Divide/1 -> Divide1/2
  y/1 -> MATLAB Function/1(u)
  Divide1/1 -> Mux/12
  MATLAB Function/1(r1) -> Mux/25
  MATLAB Function/2(r2) -> Mux/26
  MATLAB Function/3(r3) -> Mux/27
  MATLAB Function/4(r4) -> Mux/29
  MATLAB Function/5(r5) -> Mux/30
  MATLAB Function/6(r6) -> Mux/31
  MATLAB Function/7(r7) -> Mux/33
  MATLAB Function/8(r8) -> Mux/34
  MATLAB Function/9(r9) -> Mux/35
  Constant1/1 -> Mux/24, Mux/23, Mux/22, Mux/21, Mux/20, Mux/19, Mux/18, Mux/17, Mux/16, Mux/15, Mux/14, Mux/13, Mux/11, Mux/10, Mux/9, Mux/8, Mux/7, Mux/6, Mux/5, Mux/4, Mux/3, Mux/2, Mux/1, Mux/28, Mux/32, Mux/36
  Mux/1 -> Reshape/1
  Reshape/1 -> c/1

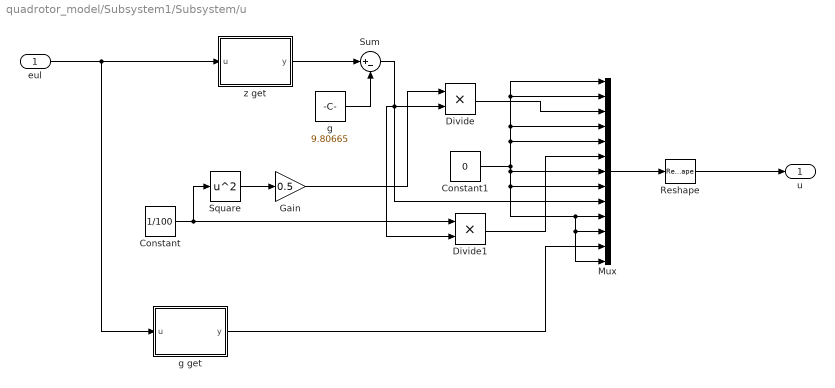
== system quadrotor_model/Subsystem1/Subsystem/u ==
  eul : Inport
  Constant : Constant  Value=1/100
  Constant1 : Constant  Value=0
  Divide : Product  Inputs=**
  Divide1 : Product  Inputs=**
  Gain : Gain  Gain=0.5
  Mux : Mux  Inputs=13
  Reshape : Reshape  OutputDimensionality=Customize  OutputDimensions=[13,1]
  Square : Math  Operator=square  SaturateOnIntegerOverflow=on
  Sum : Sum  Inputs=|+-
  g : Constant  Value=9.80665
  g get : MATLAB Function  TreatAsAtomicUnit=on
  z get : MATLAB Function  TreatAsAtomicUnit=on
  u : Outport  SampleTime=1/100
  wires:
  Constant/1 -> Divide1/1, Square/1
  Square/1 -> Gain/1
  eul/1 -> g get/1(u), z get/1(u)
  z get/1(y) -> Sum/1
  g/1 -> Sum/2
  Gain/1 -> Divide/1
  Sum/1 -> Mux/9, Divide/2, Divide1/2
  Divide/1 -> Mux/3
  Divide1/1 -> Mux/6
  g get/1(y) -> Mux/12
  Constant1/1 -> Mux/13, Mux/11, Mux/10, Mux/8, Mux/7, Mux/5, Mux/4, Mux/1, Mux/2
  Mux/1 -> Reshape/1
  Reshape/1 -> u/1

== system quadrotor_model/Subsystem1/Subsystem/y ==
  a_G : Inport
  p : Inport  Port=2
  Constant : Constant  Value=0
  Demux : Demux  Outputs=3
  Demux1 : Demux  Outputs=3
  Mux : Mux
  Terminator{,1..3} (4 alike) : Terminator
  y : Outport  SampleTime=1/100
  wires:
  a_G/1 -> Demux/1
  Demux/1 -> Terminator/1
  Demux/2 -> Terminator1/1
  Demux1/2 -> Terminator3/1
  p/1 -> Demux1/1
  Demux1/1 -> Terminator2/1
  Demux1/3 -> Mux/4
  Demux/3 -> Mux/3
  Constant/1 -> Mux/2, Mux/1
  Mux/1 -> y/1

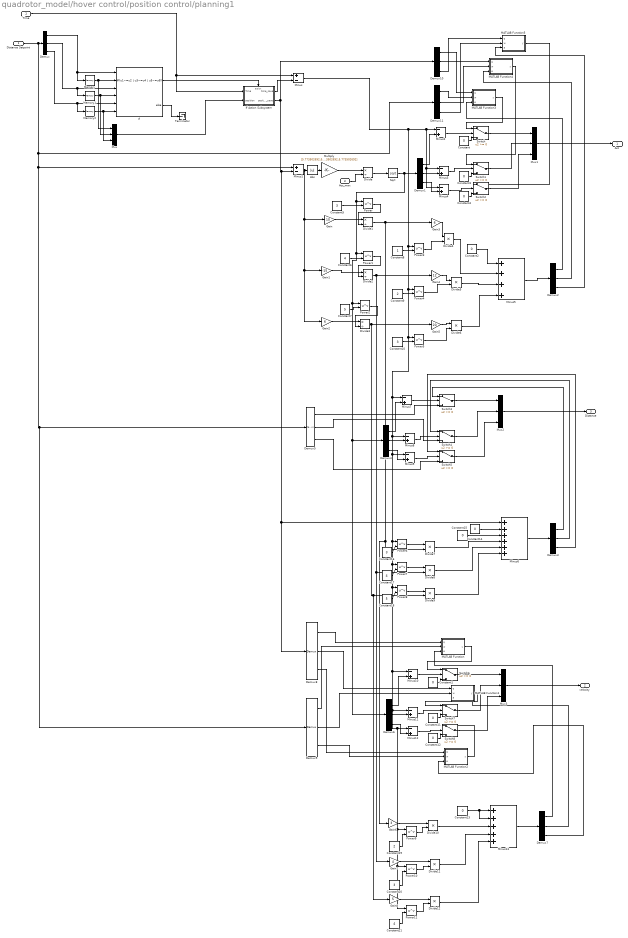
== system quadrotor_model/hover control/position control/planning1 ==
  Distance Setpoint : Inport
  Time : Inport  Port=2
  Acc_max : Inport  Port=3
  Abs : Abs
  Constant{,1..4,11..15} (10 alike) : Constant  Value=0
  Constant{5,10,16,20} (4 alike) : Constant  Value=3
  Constant17 : Constant  Value=4
  Constant18 : Constant  Value=5
  Constant19 : Constant  Value=2
  Constant21 : Constant  Value=4
  Constant6 : Constant  Value=4
  Constant7 : Constant  Value=5
  Constant8 : Constant
  Constant9 : Constant  Value=2
  Demux{,1..11} (12 alike) : Demux  Outputs=3
  Divide{,1..3} (4 alike) : Product  Inputs=*/
  Divide{4..12} (9 alike) : Product  Inputs=**
  Gain : Gain  Gain=10
  Gain1 : Gain  Gain=-15
  Gain2 : Gain  Gain=6
  Gain3 : Gain  Gain=6
  Gain4 : Gain  Gain=12
  Gain5 : Gain  Gain=20
  Gain6 : Gain  Gain=3
  Gain7 : Gain  Gain=4
  Gain8 : Gain  Gain=5
  If : If  NumInputs=6  IfExpression=(u1~=u2 | u3~=u4 | u5~=u6)
  If Action Subsystem : Subsystem  TreatAsAtomicUnit=on
  MATLAB Function : MATLAB Function  TreatAsAtomicUnit=on
  MATLAB Function1 : MATLAB Function  TreatAsAtomicUnit=on
  MATLAB Function2 : MATLAB Function  TreatAsAtomicUnit=on
  MATLAB Function3 : MATLAB Function  TreatAsAtomicUnit=on
  MATLAB Function4 : MATLAB Function  TreatAsAtomicUnit=on
  MATLAB Function5 : MATLAB Function  TreatAsAtomicUnit=on
  Memory : Memory
  Memory1 : Memory
  Memory2 : Memory
  Minus : Sum  Inputs=+-
  Minus1 : Sum  Inputs=+-
  Minus{2..4,7..12} (9 alike) : Sum  Inputs=-+
  Minus13 : Sum  Inputs=+++++
  Minus5 : Sum  Inputs=++++
  Minus6 : Sum  Inputs=++++++
  Multiply : Gain  Gain=[5.773502692;5.773502692;5.773502692]
  Mux{,1..3} (4 alike) : Mux  Inputs=3
  Power{,1..11} (12 alike) : Math  Operator=pow  SaturateOnIntegerOverflow=on
  Sqrt : Sqrt  SaturateOnIntegerOverflow=on
  Switch{,1..8} (9 alike) : Switch
  Terminator : Terminator
  "Acc " : Outport
  velocity : Outport  Port=2
  Distance : Outport  Port=3
  wires:
  If/1 -> If Action Subsystem/Action
  Memory/1 -> Mux/1, If/2
  Time/1 -> Minus/1, If Action Subsystem/1(Time)
  Demux/1 -> Memory/1, If/1
  Memory1/1 -> Mux/2, If/4
  Memory2/1 -> Mux/3, If/6
  Demux/2 -> Memory1/1, If/3
  Demux/3 -> Memory2/1, If/5
  Mux/1 -> If Action Subsystem/2(position)
  Multiply/1 -> Divide/1
  Acc_max/1 -> Divide/2
  Divide/1 -> Sqrt/1
  Constant/1 -> Switch/3
  Mux1/1 -> "Acc "/1
  Switch/1 -> Mux1/1
  Constant3/1 -> Switch1/3
  Constant4/1 -> Switch2/3
  Switch1/1 -> Mux1/2
  Switch2/1 -> Mux1/3
  Demux1/2 -> Minus3/2
  Minus3/1 -> Switch1/2
  Demux1/3 -> Minus4/2
  Minus4/1 -> Switch2/2
  Gain/1 -> Divide1/1
  Constant5/1 -> Power/2
  Power/1 -> Divide1/2
  Constant6/1 -> Power1/2
  Gain1/1 -> Divide2/1
  Power1/1 -> Divide2/2
  Constant7/1 -> Power2/2
  Demux1/1 -> Minus2/2
  Minus1/1 -> Gain1/1, Gain2/1, Gain/1, Abs/1
  Power2/1 -> Divide3/2
  Gain2/1 -> Divide3/1
  Minus5/1 -> Demux2/1
  Demux2/1 -> MATLAB Function3/3(e)
  Demux2/3 -> MATLAB Function5/3(e)
  Constant2/1 -> Minus5/1
  Gain3/1 -> Divide4/1
  Divide4/1 -> Minus5/2
  Gain4/1 -> Divide5/1
  Divide5/1 -> Minus5/3
  Gain5/1 -> Divide6/1
  Divide6/1 -> Minus5/4
  Power3/1 -> Divide4/2
  Constant8/1 -> Power3/2
  Constant9/1 -> Power4/2
  Constant10/1 -> Power5/2
  Minus2/1 -> Switch/2
  Power4/1 -> Divide5/2
  Power5/1 -> Divide6/2
  Switch5/1 -> Mux2/3
  Minus7/1 -> Switch3/2
  Demux4/1 -> Minus7/2
  Demux4/3 -> Minus9/2
  Demux3/3 -> Switch5/1
  Switch3/1 -> Mux2/1
  Demux3/2 -> Switch4/1
  Demux3/1 -> Switch3/1
  Minus9/1 -> Switch5/2
  Minus8/1 -> Switch4/2
  Demux4/2 -> Minus8/2
  Switch4/1 -> Mux2/2
  Demux5/3 -> Switch5/3
  Demux5/1 -> Switch3/3
  Demux5/2 -> Switch4/3
  Mux2/1 -> Distance/1
  Minus6/1 -> Demux3/1
  If Action Subsystem/2(position_save) -> Demux8/1, Minus6/1, Minus1/2, Demux10/1
  Constant14/1 -> Minus6/2
  Constant15/1 -> Minus6/3
  Divide7/1 -> Minus6/4
  Divide8/1 -> Minus6/5
  Divide9/1 -> Minus6/6
  Power6/1 -> Divide7/1
  Power7/1 -> Divide8/1
  Power8/1 -> Divide9/1
  Constant16/1 -> Power6/2
  Constant17/1 -> Power7/2
  Constant18/1 -> Power8/2
  Distance Setpoint/1 -> Demux9/1, Demux5/1, Minus1/1, Demux11/1, Demux/1
  Abs/1 -> Multiply/1
  Switch8/1 -> Mux3/3
  Minus10/1 -> Switch6/2
  Sqrt/1 -> Demux4/1, Demux6/1, Power2/1, Power1/1, Power/1, Demux1/1
  Demux6/1 -> Minus10/2
  Demux6/3 -> Minus12/2
  Demux7/3 -> MATLAB Function2/3(e)
  Switch6/1 -> Mux3/1
  Demux7/2 -> MATLAB Function1/3(e)
  Demux7/1 -> MATLAB Function/3(e)
  Minus/1 -> Minus4/1, Minus3/1, Minus2/1, Power3/1, Minus7/1, Power6/1, Minus10/1, Minus11/1, Power9/1, Power11/1, Power10/1, Minus12/1, Power8/1, Power7/1, Minus9/1, Minus8/1, Power5/1, Power4/1
  Minus12/1 -> Switch8/2
  Minus11/1 -> Switch7/2
  Demux6/2 -> Minus11/2
  Switch7/1 -> Mux3/2
  Constant12/1 -> Switch8/3
  Constant1/1 -> Switch6/3
  Constant11/1 -> Switch7/3
  Mux3/1 -> velocity/1
  Minus13/1 -> Demux7/1
  Constant13/1 -> Minus13/2, Minus13/1
  Divide10/1 -> Minus13/3
  Divide11/1 -> Minus13/4
  Divide12/1 -> Minus13/5
  Gain6/1 -> Divide10/1
  Gain7/1 -> Divide11/1
  Gain8/1 -> Divide12/1
  Divide1/1 -> Gain3/1, Gain6/1, Divide7/2
  Divide2/1 -> Gain4/1, Gain7/1, Divide8/2
  Divide3/1 -> Gain5/1, Gain8/1, Divide9/2
  Power9/1 -> Divide10/2
  Power11/1 -> Divide12/2
  Power10/1 -> Divide11/2
  Constant19/1 -> Power9/2
  Constant20/1 -> Power10/2
  Constant21/1 -> Power11/2
  Demux8/1 -> MATLAB Function/1(q)
  Demux9/1 -> MATLAB Function/2(w)
  MATLAB Function/1(y) -> Switch6/1
  Demux8/2 -> MATLAB Function1/1(q)
  Demux9/2 -> MATLAB Function1/2(w)
  MATLAB Function1/1(y) -> Switch7/1
  Demux8/3 -> MATLAB Function2/1(q)
  Demux9/3 -> MATLAB Function2/2(w)
  MATLAB Function2/1(y) -> Switch8/1
  Demux10/1 -> MATLAB Function3/1(q)
  Demux11/1 -> MATLAB Function3/2(w)
  Demux10/2 -> MATLAB Function4/1(q)
  Demux11/2 -> MATLAB Function4/2(w)
  Demux2/2 -> MATLAB Function4/3(e)
  MATLAB Function4/1(y) -> Switch1/1
  Demux11/3 -> MATLAB Function5/2(w)
  Demux10/3 -> MATLAB Function5/1(q)
  MATLAB Function5/1(y) -> Switch2/1
  If Action Subsystem/1("time_save ") -> Minus/2
  MATLAB Function3/1(y) -> Switch/1
  If/2 -> Terminator/1

== system quadrotor_model/hover control/position control/planning1/If Action Subsystem ==
  Time : Inport
  position : Inport  Port=2
  Action Port : ActionPort  InitializeStates=reset  PropagateVarSize=During execution  ActionPortLabel=if((u1~=u2 | u3~=u4 | u5~=u6))
  "time_save " : Outport
  position_save : Outport  Port=2
  wires:
  Time/1 -> "time_save "/1
  position/1 -> position_save/1

== matlab function quadrotor_model/hover control/position control/planning1/MATLAB Function1 ==
  data: q input; y output; w input; e input
function y = fcn(q,w,e)
  if(q==w)
    y=0;
  else 
    y = e; 
  end

end

== matlab function quadrotor_model/hover control/position control/planning1/MATLAB Function2 ==
  data: q input; y output; w input; e input
function y = fcn(q,w,e)
  if(q==w)
    y=0;
  else 
    y = e; 
  end

end

== matlab function quadrotor_model/hover control/position control/planning1/MATLAB Function3 ==
  data: q input; y output; w input; e input
function y = fcn(q,w,e)
  if(q==w)
    y=0;
  else 
    y = e; 
  end

end

== matlab function quadrotor_model/hover control/position control/planning1/MATLAB Function4 ==
  data: q input; y output; w input; e input
function y = fcn(q,w,e)
  if(q==w)
    y=0;
  else 
    y = e; 
  end

end

== matlab function quadrotor_model/hover control/position control/planning1/MATLAB Function5 ==
  data: q input; y output; w input; e input
function y = fcn(q,w,e)
  if(q==w)
    y=0;
  else 
    y = e; 
  end

end

== matlab function quadrotor_model/hover control/position control/MATLAB Function ==
  data: u input; y output
function y = checkNan(u)
if isnan(u(1))
    u(1) = 0;
end
if isnan(u(2))
    u(2) = 0;
end
if isnan(u(3))
    u(3) = 0;
end
        
y = u;

== matlab function quadrotor_model/Quadrotor/MATLAB Function ==
  data: u input; y output
function y = quat2Rom(u)

y = quat2rotm(u');

== matlab function quadrotor_model/hover control/Desire Angle/MATLAB Function2 ==
  data: u input; y output
function y = checkNan(u)
if isnan(u(1)) || isinf(u(1))
    u(1) = 0;
end
if isnan(u(2)) || isinf(u(2))
    u(2) = 0;
end
if isnan(u(3)) || isinf(u(3))
    u(3) = 0;
end
        
y = u;

== matlab function quadrotor_model/Quadrotor/quat2Rotm2/MATLAB Function ==
  data: u input; y output
function y = skewOperator(u)

y =[0 -u(3) u(2) ; u(3) 0 -u(1) ; -u(2) u(1) 0 ];

== matlab function quadrotor_model/hover control/MATLAB Function ==
  data: u input; y output
function y = checkNan(u)
if isnan(u(1))
    u(1) = 0;
end
if isnan(u(2))
    u(2) = 0;
end
if isnan(u(3))
    u(3) = 0;
end
        
y = u;

== matlab function quadrotor_model/Subsystem1/Subsystem/euler ==
  data: u input; y output
function y  = fcn(u)

y = eul2rotm(u);

== matlab function quadrotor_model/Subsystem1/Subsystem/u/z get ==
  data: u input; y output
function y = fcn(u)
 u = u*[0 0 1]'
y = u(3);

== matlab function quadrotor_model/Subsystem1/Subsystem/c/MATLAB Function ==
  data: u input; r1 output; r2 output; r3 output; r4 output; r5 output; r6 output; r7 output; r8 output; r9 output
function [r1,r2,r3,r4,r5,r6,r7,r8,r9] = fcn(u)
 r1 = u(1,1)  
 r2 = u(1,2)
 r3 = u(1,3)
 r4 = u(2,1)
 r5 = u(2,2) 
 r6 = u(2,3)
 r7 = u(3,1)
 r8 = u(3,2)
 r9 = u(3,3)

== matlab function quadrotor_model/Subsystem1/Subsystem/u/g get ==
  data: u input; y output
function y = fcn(u)
u = u*[0 0 -9.80665]'
y = u(3);

== matlab function quadrotor_model/hover control/Subsystem/MATLAB Function ==
  data: r input; q output
function q = eulerToQuaternion(r)
    
q = eul2quat(r);

== matlab function quadrotor_model/hover control/position control/planning1/MATLAB Function ==
  data: q input; y output; w input; e input
function y = fcn(q,w,e)
  if(q==w)
    y=0;
  else 
    y = e; 
  end

end
